simulink model "ES229A_HwTqCorrln"  (R2013b)
settings: Solver=FixedStepDiscrete  SolverMode=SingleTasking  StartTime=0.0  StopTime=1  FixedStep=0.002  RelTol=1e-3
undefined symbols (not defined in the file): ARCHGLBPRM_100MILLISEC_SEC_F32, FLTINJ_HWTQCORRLN_HWTQIDPTSIG, HwTqCorrlnChACmnModCmpLpFilActvnThd, HwTqCorrlnChACmnModCmpLpFilOutpLim, HwTqCorrlnChAImdtCorrlnChkFailThd, HwTqCorrlnChAImdtCorrlnChkPassThd, HwTqCorrlnChAStabStClrFltThd, HwTqCorrlnChAStabStSetFltThd, HwTqCorrlnChATqSumMaxLim, HwTqCorrlnChATraSumClrFltThd, HwTqCorrlnChATraSumSetFltThd, HwTqCorrlnChBCmnModCmpLpFilActvnThd, HwTqCorrlnChBCmnModCmpLpFilOutpLim, HwTqCorrlnChBImdtCorrlnChkFailThd, HwTqCorrlnChBImdtCorrlnChkPassThd, HwTqCorrlnChBStabStClrFltThd, HwTqCorrlnChBStabStSetFltThd, HwTqCorrlnChBTqSumMaxLim, HwTqCorrlnChBTraSumClrFltThd, HwTqCorrlnChBTraSumSetFltThd, HwTqCorrlnMaxStallTqA, HwTqCorrlnMaxStallTqB, HwTqCorrlnMaxStallTqC, HwTqCorrlnMaxStallTqD, HWTQSCA_CNT_U08, NtcNr1, NtcSts1, PARAMETERBYTE_CNT_U08, sigbuilder_block, SigQlfr1, STABSTLPFILSTVARIDELTALIM_HWNWTMTR_F32
libraries: simulink x25, Fil x12, NxtrLim x10, NxtrAbslt x6, FixdToFloat x2, FloatToFixdWithRound x2, LnrIntrpn x2, NxtrNvM x2
(part 1 of 4)
settings Model: Creator=nzy7l3  LastModifiedBy=CZ68DS
settings SolverCC: AutoInsertRateTranBlk=on  InsertRTBMode=Always
settings DataIOCC: LimitDataPoints=off  SaveFormat=Structure  ReturnWorkspaceOutputs=on
settings OptimizationCC: BlockReduction=off  InlineParams=on  ZeroExternalMemoryAtStartup=off  ZeroInternalMemoryAtStartup=off  OptimizeModelRefInitCode=on  LifeSpan=1
settings DebuggingCC: SignalInfNanChecking=error  SignalRangeChecking=warning  UnderspecifiedInitializationDetection=Simplified  MergeDetectMultiDrivingBlocksExec=error  SolverPrmCheckMsg=error  InheritedTsInSrcMsg=error  SingleTaskRateTransMsg=error  TasksWithSamePriorityMsg=error  SigSpecEnsureSampleTimeMsg=error  CheckMatrixSingularityMsg=error  ParameterUnderflowMsg=error  ParameterPrecisionLossMsg=error  ParameterTunabilityLossMsg=error  FixptConstUnderflowMsg=warning  FixptConstOverflowMsg=warning  VectorMatrixConversionMsg=error  SignalLabelMismatchMsg=error  UnconnectedInputMsg=error  UnconnectedOutputMsg=error  UnconnectedLineMsg=error  SFcnCompatibilityMsg=error  FrameProcessingCompatibilityMsg=error  UniqueDataStoreMsg=warning  BusObjectLabelMismatch=error  RootOutportRequireBusObject=error  AssertControl=DisableAll  ModelReferenceIOMsg=error  ModelReferenceVersionMismatchMessage=warning  ModelReferenceIOMismatchMessage=error  ModelReferenceDataLoggingMessage=error  StateNameClashWarn=warning  StrictBusMsg=ErrorOnBusTreatedAsVector  NonBusSignalsTreatedAsBus=error  SFUnexpectedBacktrackingDiag=error  SFInvalidInputDataAccessInChartInitDiag=error  SFNoUnconditionalDefaultTransitionDiag=error  SFTransitionOutsideNaturalParentDiag=error  SFUnconditionalTransitionShadowingDiag=error  SFUndirectedBroadcastEventsDiag=error
settings ModelReferenceCC: ModelReferenceNumInstancesAllowed=Single
settings RTWCC: SystemTargetFile=autosar.tlc  GenCodeOnly=on  TemplateMakefile=ert_default_tmf  Description=AUTOSAR  GenerateReport=on  LaunchReport=on
settings CodeAppCC: GenerateComments=off  IgnoreCustomStorageClasses=off  CustomSymbolStrType=$N$R$M  CustomSymbolStrBlkIO=$N$M  SimulinkBlockComments=off
settings STFCustomTargetCC: CodeReplacementLibrary=C89/C90 (ANSI)  ParMdlRefBuildCompliant=on  CompOptLevelCompliant=on  IncludeMdlTerminateFcn=off  CombineOutputUpdateFcns=on  SuppressErrorStatus=on  ERTFirstTimeCompliant=on  ERTCustomFileBanners=on  SupportNonFinite=off  SupportComplex=off  SupportContinuousTime=off  SupportNonInlinedSFcns=off  MATLABClassNameForMDSCustomization=Simulink.SoftwareTarget.ERTCustomization  AutosarCompliant=on  GRTInterface=off  SystemTargetFile=autosar.tlc
settings ERTTargetCC: CodeReplacementLibrary=C89/C90 (ANSI)  ConcurrentExecutionCompliant=off  IncludeMdlTerminateFcn=off  SuppressErrorStatus=on  SupportNonFinite=off  SupportComplex=off  ModelStepFunctionPrototypeControlCompliant=off  CPPClassGenCompliant=off  AutosarCompliant=on  InlinedParameterPlacement=NonHierarchical  ERTCustomFileTemplate=example_file_process.tlc  EnableUserReplacementTypes=on

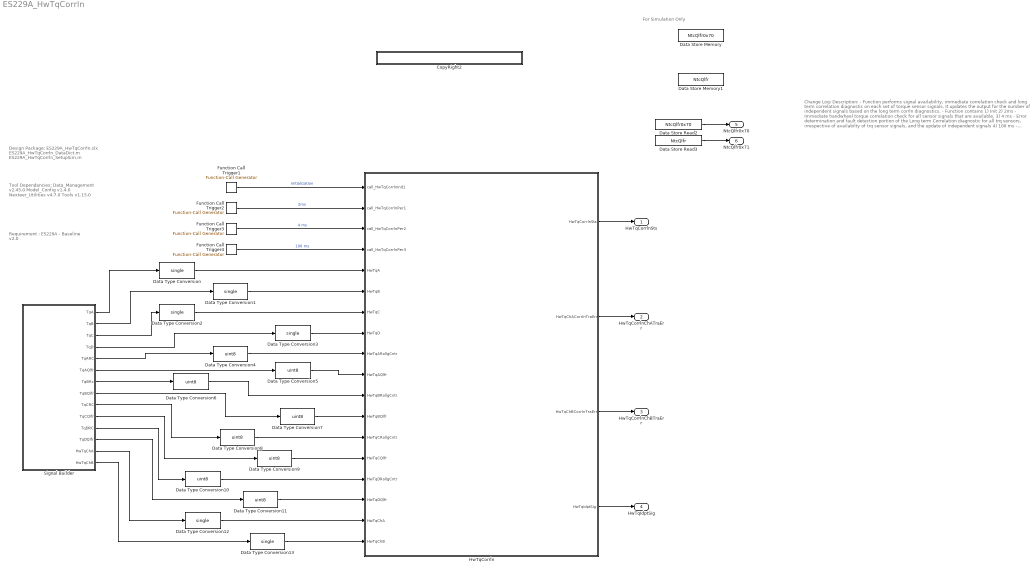
== system ES229A_HwTqCorrln ==
  note: Change Log:
      |
      | Description:
      | - Function performs signal availability, immediate correlation check and long term correlation diagnostic
      | on each set of torque sensor signals.
      | It updates the output for the number of independent signals based on the long term corrln diagnostics.
      | - Function contains
      | 1) Init
      | 2) 2ms - Immediate handwheel torque correlation check for all sensor signals that are available.
      | 3) 4 ms - Error determination and fault detection portion of the Long term Correlation diagnostic for all trq sensors,
      | irrespective of availabilty of trq sensor signals, and the update of independent signals
      | 4) 100 ms - Common mode long term compensation component of the Correlation diagnostic based on trimmed hw tq
      | derived from a pair of trq sensors.
      |
      | Copyright Blocks added to each layer
      |
      |
      | Rev: 3.2.0
      | Date:12OCT2016
      | Change Control #: EA4#8002
      | DRW: Keyur Patel
      | Description:
      | Code Impact:
      | - corrected FLTINJ_HWTQCORRLN_HWTQIDPTSIG as per DF001A
      |
      |
      | Rev: 3.1.0
      | Date:12SEPT2016
      | Change Control #: EA4#7556
      | DRW: Keyur Patel
      | Description:
      | Code Impact:
      | - Use     instead of FLTINJ_IDPTSIG_HWTQCORRLN in m file.
      |
      | Rev: 3.0.0
      | Date:28MAR2016
      | Change Control #: EA4#5051, EA4#5018
      | DRW: Praveen Devaraj / Muragesh Asundi (KPIT)
      | Description:
      | Code Impact:
      | - Two output variables HwTqChACorrlnTraErr and HwTqChBCorrlnTraErr have been added
      | -  Limit function is also added for these outputs
      | - Display variables 'dHwTqCorrlnChATraErr' and 'dHwTqCorrlnChBTraErr' have been deleted
      | No Code Impact:
      | - As per Anomaly  EA4#2139, model clean up is done function 'HwTqCorrlnInit1' to match code.
      | Color code:
      | - All changes are highlighted in red foreground color
      |
      | Rev: Synergy
      | Date:27OCT2015
      | Change Control #: EA4#2119
      | DRW: A.Amberkar
      | Description:
      | - Captured in WR comments - NtcNr2 revise to NtcNr1 and use LimDyn_f32 library block.
      | - For anomaly#2139 to prepare model for MIL testing - removed delay blocks in Signal availability
      | and replaced with already defined PIM data.
      |
      | Rev: Synergy
      | Date:01OCT2015
      | Change Control #: EA4#1347
      | DRW: A.Amberkar
      | Description:
      | - Captured in WR comments - new immdt corrln check, limit on SS LPF, new independent signals truth table
      |
      | Rev: Synergy
      | Date: 11AUG2015
      | Change Control #:EA4#1273
      | DRW: A.Amberkar
      | Description:
      | - Changes to match code - captured in WR comments
      |
      | Rev: Synergy
      | Date: 13JUL2015
      | Change Control #:EA4#768
      | DRW: A.Amberkar
      | Description:
      | - Initial Release
      |
      | Rev: Synergy
      | Date: 17JUN2015
      | Change Control #: EA4#768
      | DRW: Aparna Amberkar
  note: Design Package:
      | ES229A_HwTqCorrln.slx
      | ES229A_HwTqCorrln_DataDict.m
      | ES229A_HwTqCorrln_SetupSim.m
  note: Tool Dependancies:
      |
      | Data_Management v2.45.0
      | Model_Config v1.4.0
      | Nexteer_Utilities v4.7.0
      | Tools v1.15.0
  note: Requirement :
      |
      | ES229A - Baseline v2.0
  note: For Simulation Only
  CopyRight2 : Subsystem  Description=|  mask(Copyright Information){none=on}
      | Copyright info block.                                               
      |                                                                     
      | Place copyright information at the top of every subsystem in design.
      mask prompts: none "No parameters"
      mask help: Place copyright information at the top of every subsystem in design.
      mask Display:
      | NxtrConf = 'Nexteer Confidential';
      | 
      | sys = bdroot; %handle for the current model ("system")
      | first = get_param(sys,'Created');
      | first = first(end-3:end);  %year is last four digits
      | 
      | last = get_param(sys,'LastModifiedDate');
      | if isempty(last)
      |     last = datestr(now,'yyyy');
      | else
      |     last = last(end-3:end);
      | end
      | 
      | if strcmp(first,last)
      |     fprintf('%s -- Copyright %s Nexteer',NxtrConf,first)
      | else
      |     fprintf('%s -- %s%s- %s Nexteer',NxtrConf,char(169),first,last)
      | end
  Data Store Read2 : DataStoreRead  DataStoreName=NtcQlfr0x70  SampleTime=.002
  Data Store Read3 : DataStoreRead  DataStoreName=NtcQlfr  SampleTime=.002
  Data Store Memory : DataStoreMemory  DataStoreName=NtcQlfr0x70  ReadBeforeWriteMsg=warning  WriteAfterWriteMsg=warning  WriteAfterReadMsg=warning  OutDataTypeStr=uint8
      settings: AttributesFormatString=|
      | Simulation Purpose Only.
      | Do Not Code this block
      | Diagnostic Manager Owns this requirement
  Data Store Memory1 : DataStoreMemory  DataStoreName=NtcQlfr  ReadBeforeWriteMsg=warning  WriteAfterWriteMsg=warning  WriteAfterReadMsg=warning  OutDataTypeStr=uint8
      settings: AttributesFormatString=|
      | Simulation Purpose Only.
      | Do Not Code this block
      | Diagnostic Manager Owns this requirement
  Data Type Conversion{,1..3,12..13} (6 alike) : DataTypeConversion  OutDataTypeStr=single
  Data Type Conversion{4..11} (8 alike) : DataTypeConversion  OutDataTypeStr=uint8
  Function Call Trigger{1..4} (4 alike) : simulink/Ports & Subsystems/Function-Call Generator  sample_time=.002  numberOfIterations=1
  HwTqCorrln : Subsystem
  Signal Builder : Subsystem  Tag=STV Subsys  LoadFcn=sigbuilder_block('load');  StartFcn=sigbuilder_block('start');  StopFcn=sigbuilder_block('stop');  ClipboardFcn=sigbuilder_block('clipboard');  mask(Sigbuilder block){}
      mask help: Simulink:masks:SigbuilderBlock_MD
      mask init:
      | if ~strcmp(get_param(bdroot(gcbh),'SimulationStatus'),'stopped') tuvar = sigbuilder_block('maskInit'); end
      settings: CopyFcn=sigbuilder_block('copy');  DeleteFcn=sigbuilder_block('delete');  ModelCloseFcn=sigbuilder_block('modelClose');  PreSaveFcn=sigbuilder_block('preSave');  PauseFcn=sigbuilder_block('pause');  ContinueFcn=sigbuilder_block('continue');  NameChangeFcn=sigbuilder_block('namechange');  OpenFcn=sigbuilder_block('open',[5.58621 28.5517 1009.24 486 ]);  CloseFcn=sigbuilder_block('close');
      mask Display: plot(0, 0, 100, 100,[2, 2, 32, 32, 2], [68, 8, 8, 68, 68],[32, 2], [38, 38], [32, 19, 2],[53, 60, 44], [32, 17, 17, 2],[16, 16, 31, 31]);txt = getActiveGroup(gcbh);text(2, 100, txt,'verticalAlignment', 'top');
  HwTqCorrlnSts : Outport
  HwTqCorrlnChATraErr : Outport  Port=2
  HwTqCorrlnChBTraErr : Outport  Port=3
  HwTqIdptSig : Outport  Port=4
  NtcQlfr0x70 : Outport  Port=5
  NtcQlfr0x71 : Outport  Port=6
  wires:
  Function Call Trigger1/1 -> HwTqCorrln/1(call_HwTqCorrlnInit1)  "Initialization"
  Function Call Trigger3/1 -> HwTqCorrln/3("call_HwTqCorrlnPer2 ")  "4 ms"
  Function Call Trigger2/1 -> HwTqCorrln/2(call_HwTqCorrlnPer1)  "2ms"
  Function Call Trigger4/1 -> HwTqCorrln/4(call_HwTqCorrlnPer3)  "100 ms"
  Signal Builder/13(HwTqChA) -> Data Type Conversion12/1
  Signal Builder/14(HwTqChB) -> Data Type Conversion13/1
  Data Type Conversion/1 -> HwTqCorrln/5(HwTqA)
  Data Type Conversion1/1 -> HwTqCorrln/6(HwTqB)
  Signal Builder/3(TqC) -> Data Type Conversion2/1
  Signal Builder/5(TqARC) -> Data Type Conversion4/1
  Signal Builder/6(TqAQlfr) -> Data Type Conversion5/1
  Signal Builder/7(TqBRc) -> Data Type Conversion6/1
  Signal Builder/8(TqBQlfr) -> Data Type Conversion7/1
  Signal Builder/9(TqCRC) -> Data Type Conversion8/1
  Signal Builder/10(TqCQlfr) -> Data Type Conversion9/1
  Signal Builder/11(TqDRC) -> Data Type Conversion10/1
  Signal Builder/12(TqDQlfr) -> Data Type Conversion11/1
  Data Type Conversion2/1 -> HwTqCorrln/7(HwTqC)
  Data Type Conversion3/1 -> HwTqCorrln/8(HwTqD)
  Data Type Conversion4/1 -> HwTqCorrln/9(HwTqARollgCntr)
  Data Type Conversion5/1 -> HwTqCorrln/10(HwTqAQlfr)
  Data Type Conversion6/1 -> HwTqCorrln/11(HwTqBRollgCntr)
  Data Type Conversion7/1 -> HwTqCorrln/12(HwTqBQlfr)
  Data Type Conversion8/1 -> HwTqCorrln/13(HwTqCRollgCntr)
  Data Type Conversion9/1 -> HwTqCorrln/14(HwTqCQlfr)
  Data Type Conversion10/1 -> HwTqCorrln/15(HwTqDRollgCntr)
  Data Type Conversion11/1 -> HwTqCorrln/16(HwTqDQlfr)
  Data Type Conversion12/1 -> HwTqCorrln/17(HwTqChA)
  Data Type Conversion13/1 -> HwTqCorrln/18(HwTqChB)
  Signal Builder/1(TqA) -> Data Type Conversion/1
  Signal Builder/2(TqB) -> Data Type Conversion1/1
  Signal Builder/4(TqD) -> Data Type Conversion3/1
  HwTqCorrln/1(HwTqCorrlnSts) -> HwTqCorrlnSts/1
  HwTqCorrln/4(HwTqIdptSig) -> HwTqIdptSig/1
  HwTqCorrln/3(HwTqChBCorrlnTraErr) -> HwTqCorrlnChBTraErr/1
  HwTqCorrln/2(HwTqChACorrlnTraErr) -> HwTqCorrlnChATraErr/1
  Data Store Read2/1 -> NtcQlfr0x70/1
  Data Store Read3/1 -> NtcQlfr0x71/1

== system ES229A_HwTqCorrln/CopyRight2 ==

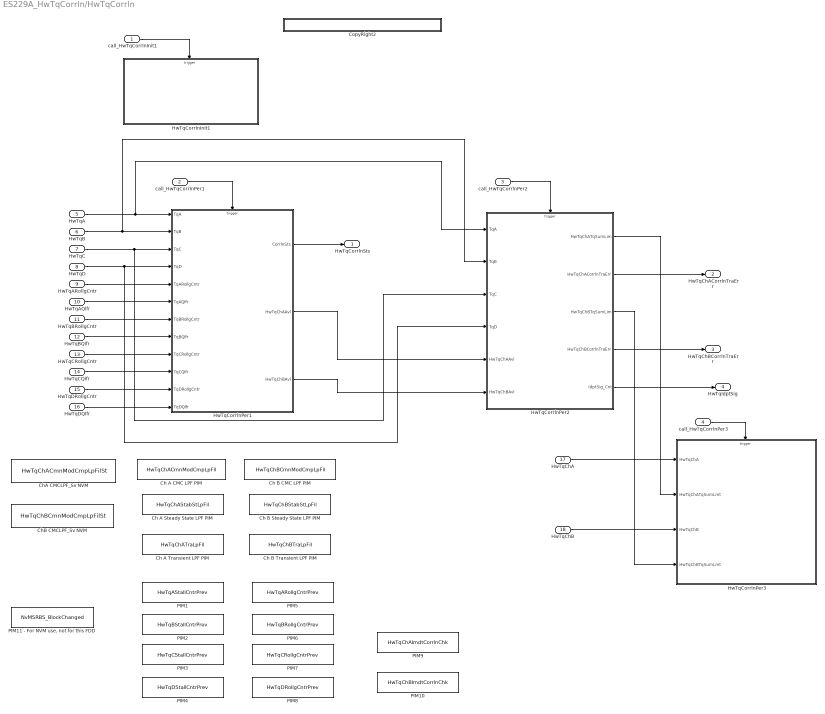
== system ES229A_HwTqCorrln/HwTqCorrln ==
  call_HwTqCorrlnInit1 : Inport
  call_HwTqCorrlnPer1 : Inport  Port=2
  "call_HwTqCorrlnPer2 " : Inport  Port=3
  call_HwTqCorrlnPer3 : Inport  Port=4
  HwTqA : Inport  Port=5
  HwTqB : Inport  Port=6
  HwTqC : Inport  Port=7
  HwTqD : Inport  Port=8
  HwTqARollgCntr : Inport  Port=9
  HwTqAQlfr : Inport  Port=10
  HwTqBRollgCntr : Inport  Port=11
  HwTqBQlfr : Inport  Port=12
  HwTqCRollgCntr : Inport  Port=13
  HwTqCQlfr : Inport  Port=14
  HwTqDRollgCntr : Inport  Port=15
  HwTqDQlfr : Inport  Port=16
  HwTqChA : Inport  Port=17
  HwTqChB : Inport  Port=18
  " PIM1" : DataStoreMemory  DataStoreName=HwTqAStallCntrPrev  ReadBeforeWriteMsg=warning  WriteAfterWriteMsg=warning  WriteAfterReadMsg=warning  StateMustResolveToSignalObject=on
  " PIM11 - For NVM use, not for this FDD" : DataStoreMemory  DataStoreName=NvMSRBS_BlockChanged  ReadBeforeWriteMsg=warning  WriteAfterWriteMsg=warning  WriteAfterReadMsg=warning
  " PIM2" : DataStoreMemory  DataStoreName=HwTqBStallCntrPrev  ReadBeforeWriteMsg=warning  WriteAfterWriteMsg=warning  WriteAfterReadMsg=warning  StateMustResolveToSignalObject=on
  " PIM3" : DataStoreMemory  DataStoreName=HwTqCStallCntrPrev  ReadBeforeWriteMsg=warning  WriteAfterWriteMsg=warning  WriteAfterReadMsg=warning  StateMustResolveToSignalObject=on
  " PIM4" : DataStoreMemory  DataStoreName=HwTqDStallCntrPrev  ReadBeforeWriteMsg=warning  WriteAfterWriteMsg=warning  WriteAfterReadMsg=warning  StateMustResolveToSignalObject=on
  " PIM5" : DataStoreMemory  DataStoreName=HwTqARollgCntrPrev  ReadBeforeWriteMsg=warning  WriteAfterWriteMsg=warning  WriteAfterReadMsg=warning  StateMustResolveToSignalObject=on
  " PIM6" : DataStoreMemory  DataStoreName=HwTqBRollgCntrPrev  ReadBeforeWriteMsg=warning  WriteAfterWriteMsg=warning  WriteAfterReadMsg=warning  StateMustResolveToSignalObject=on
  " PIM7" : DataStoreMemory  DataStoreName=HwTqCRollgCntrPrev  ReadBeforeWriteMsg=warning  WriteAfterWriteMsg=warning  WriteAfterReadMsg=warning  StateMustResolveToSignalObject=on
  " PIM8" : DataStoreMemory  DataStoreName=HwTqDRollgCntrPrev  ReadBeforeWriteMsg=warning  WriteAfterWriteMsg=warning  WriteAfterReadMsg=warning  StateMustResolveToSignalObject=on
  " PIM9" : DataStoreMemory  DataStoreName=HwTqChAImdtCorrlnChk  ReadBeforeWriteMsg=warning  WriteAfterWriteMsg=warning  WriteAfterReadMsg=warning  StateMustResolveToSignalObject=on
  Ch A CMC LPF PIM : DataStoreMemory  RequirementInfo="{'linktype_rmi_doors' '0000c477 (/ESG Group/FDD Module Requirements/EA4 Specific/ES229A_HwTqCorrln)' '#ES229A_123' 'true' 'REQ:  ES229A_123' '' } %GIDa_6766c665_50e1_4b65_9ecd_d704019af802"  DataStoreName=HwTqChACmnModCmpLpFil  ReadBeforeWriteMsg=warning  WriteAfterWriteMsg=warning  WriteAfterReadMsg=warning  InitialValue=struct('FilSt',single(0),'FilGain',single(0))  OutDataTypeStr=Bus: FilLpRec1  StateMustResolveToSignalObject=on
  Ch A Steady State LPF PIM : DataStoreMemory  RequirementInfo="{'linktype_rmi_doors' '0000c477 (/ESG Group/FDD Module Requirements/EA4 Specific/ES229A_HwTqCorrln)' '#ES229A_118' 'true' 'REQ:  ES229A_118' '' } %GIDa_9e19175a_f7a8_42e9_9550_54226049f41b"  DataStoreName=HwTqChAStabStLpFil  ReadBeforeWriteMsg=warning  WriteAfterWriteMsg=warning  WriteAfterReadMsg=warning  InitialValue=struct('FilSt',single(0),'FilGain',single(0))  OutDataTypeStr=Bus: FilLpRec1  StateMustResolveToSignalObject=on
  Ch A Transient LPF PIM : DataStoreMemory  RequirementInfo="{'linktype_rmi_doors' '0000c477 (/ESG Group/FDD Module Requirements/EA4 Specific/ES229A_HwTqCorrln)' '#ES229A_117' 'true' 'REQ:  ES229A_117' '' } %GIDa_8850e544_67f8_4526_8ea6_263e9ece6630"  DataStoreName=HwTqChATraLpFil  ReadBeforeWriteMsg=warning  WriteAfterWriteMsg=warning  WriteAfterReadMsg=warning  InitialValue=struct('FilSt',single(0),'FilGain',single(0))  OutDataTypeStr=Bus: FilLpRec1  StateMustResolveToSignalObject=on
  Ch B CMC LPF PIM : DataStoreMemory  RequirementInfo="{'linktype_rmi_doors' '0000c477 (/ESG Group/FDD Module Requirements/EA4 Specific/ES229A_HwTqCorrln)' '#ES229A_133' 'true' 'REQ:  ES229A_133' '' } %GIDa_5dd4475c_8cba_4d1f_98d6_68220c356134"  DataStoreName=HwTqChBCmnModCmpLpFil  ReadBeforeWriteMsg=warning  WriteAfterWriteMsg=warning  WriteAfterReadMsg=warning  InitialValue=struct('FilSt',single(0),'FilGain',single(0))  OutDataTypeStr=Bus: FilLpRec1  StateMustResolveToSignalObject=on
  Ch B Steady State LPF PIM : DataStoreMemory  RequirementInfo="{'linktype_rmi_doors' '0000c477 (/ESG Group/FDD Module Requirements/EA4 Specific/ES229A_HwTqCorrln)' '#ES229A_132' 'true' 'REQ:  ES229A_132' '' } %GIDa_17cd5088_b902_4a38_b561_38fb02043e47"  DataStoreName=HwTqChBStabStLpFil  ReadBeforeWriteMsg=warning  WriteAfterWriteMsg=warning  WriteAfterReadMsg=warning  InitialValue=struct('FilSt',single(0),'FilGain',single(0))  OutDataTypeStr=Bus: FilLpRec1  StateMustResolveToSignalObject=on
  Ch B Transient LPF PIM : DataStoreMemory  RequirementInfo="{'linktype_rmi_doors' '0000c477 (/ESG Group/FDD Module Requirements/EA4 Specific/ES229A_HwTqCorrln)' '#ES229A_131' 'true' 'REQ:  ES229A_131' '' } %GIDa_8ffac466_7c6f_4ce2_8da4_58b961cf122e"  DataStoreName=HwTqChBTraLpFil  ReadBeforeWriteMsg=warning  WriteAfterWriteMsg=warning  WriteAfterReadMsg=warning  InitialValue=struct('FilSt',single(0),'FilGain',single(0))  OutDataTypeStr=Bus: FilLpRec1  StateMustResolveToSignalObject=on
  "ChA CMCLPF_Sv NVM " : DataStoreMemory  RequirementInfo="{'linktype_rmi_doors' '0000c477 (/ESG Group/FDD Module Requirements/EA4 Specific/ES229A_HwTqCorrln)' '#ES229A_108' 'true' 'REQ:  ES229A_108' '' } %GIDa_3034ba17_e21f_4c4f_92c6_2686ce98dd15"  DataStoreName=HwTqChACmnModCmpLpFilSt  ReadBeforeWriteMsg=warning  WriteAfterWriteMsg=warning  WriteAfterReadMsg=warning  StateMustResolveToSignalObject=on
  ChB CMCLPF_Sv NVM : DataStoreMemory  RequirementInfo="{'linktype_rmi_doors' '0000c477 (/ESG Group/FDD Module Requirements/EA4 Specific/ES229A_HwTqCorrln)' '#ES229A_109' 'true' 'REQ:  ES229A_109' '' } %GIDa_0d493052_0847_4007_805a_59667ab2ab4a"  DataStoreName=HwTqChBCmnModCmpLpFilSt  ReadBeforeWriteMsg=warning  WriteAfterWriteMsg=warning  WriteAfterReadMsg=warning  StateMustResolveToSignalObject=on
  CopyRight2 : Subsystem  Description=|  mask(Copyright Information){none=on}
      | Copyright info block.                                               
      |                                                                     
      | Place copyright information at the top of every subsystem in design.
      mask prompts: none "No parameters"
      mask help: Place copyright information at the top of every subsystem in design.
      mask Display:
      | NxtrConf = 'Nexteer Confidential';
      | 
      | sys = bdroot; %handle for the current model ("system")
      | first = get_param(sys,'Created');
      | first = first(end-3:end);  %year is last four digits
      | 
      | last = get_param(sys,'LastModifiedDate');
      | if isempty(last)
      |     last = datestr(now,'yyyy');
      | else
      |     last = last(end-3:end);
      | end
      | 
      | if strcmp(first,last)
      |     fprintf('%s -- Copyright %s Nexteer',NxtrConf,first)
      | else
      |     fprintf('%s -- %s%s- %s Nexteer',NxtrConf,char(169),first,last)
      | end
  HwTqCorrlnInit1 : Subsystem  TreatAsAtomicUnit=on
  HwTqCorrlnPer1 : Subsystem  RequirementInfo={} %GIDa_553bcabc_51d1_46d6_b172_9c866a2e5d81  TreatAsAtomicUnit=on
  HwTqCorrlnPer2 : Subsystem  RequirementInfo={} %GIDa_3a71e2f5_a14f_415b_8a15_f21caafb563d  TreatAsAtomicUnit=on
  HwTqCorrlnPer3 : Subsystem  TreatAsAtomicUnit=on
  PIM10 : DataStoreMemory  DataStoreName=HwTqChBImdtCorrlnChk  ReadBeforeWriteMsg=warning  WriteAfterWriteMsg=warning  WriteAfterReadMsg=warning  StateMustResolveToSignalObject=on
  HwTqCorrlnSts : Outport
  HwTqChACorrlnTraErr : Outport  RequirementInfo={'linktype_rmi_doors' '0000c477 (/ESG Group/FDD Module Requirements/EA4 Specific/ES229A_HwTqCorrln)' '#ES229A_165' 'true' 'REQ: ES229A_165' '' } %GIDa_67389848_7ddc_4db7_86e8_1b151ddb89f7  Port=2
  HwTqChBCorrlnTraErr : Outport  RequirementInfo={'linktype_rmi_doors' '0000c477 (/ESG Group/FDD Module Requirements/EA4 Specific/ES229A_HwTqCorrln)' '#ES229A_166' 'true' 'REQ: ES229A_166' '' } %GIDa_a2392685_2b71_4620_85c8_5b6a06a62cb6  Port=3
  HwTqIdptSig : Outport  Port=4
  wires:
  call_HwTqCorrlnInit1/1 -> HwTqCorrlnInit1/Trigger
  call_HwTqCorrlnPer1/1 -> HwTqCorrlnPer1/Trigger
  "call_HwTqCorrlnPer2 "/1 -> HwTqCorrlnPer2/Trigger
  HwTqCorrlnPer1/1(CorrlnSts) -> HwTqCorrlnSts/1
  call_HwTqCorrlnPer3/1 -> HwTqCorrlnPer3/Trigger
  HwTqCorrlnPer2/5(IdptSig_Cnt) -> HwTqIdptSig/1
  HwTqCorrlnPer2/1(HwTqChATqSumLim) -> HwTqCorrlnPer3/2(HwTqChATqSumLmt)
  HwTqChA/1 -> HwTqCorrlnPer3/1(HwTqChA)
  HwTqChB/1 -> HwTqCorrlnPer3/3(HwTqChB)
  HwTqAQlfr/1 -> HwTqCorrlnPer1/6(TqAQlfr)
  HwTqA/1 -> HwTqCorrlnPer2/1(TqA), HwTqCorrlnPer1/1(TqA)
  HwTqB/1 -> HwTqCorrlnPer2/2(TqB), HwTqCorrlnPer1/2(TqB)
  HwTqC/1 -> HwTqCorrlnPer1/3(TqC), HwTqCorrlnPer2/3(TqC)
  HwTqD/1 -> HwTqCorrlnPer2/4(TqD), HwTqCorrlnPer1/4(TqD)
  HwTqARollgCntr/1 -> HwTqCorrlnPer1/5(TqARollgCntr)
  HwTqBRollgCntr/1 -> HwTqCorrlnPer1/7(TqBRollgCntr)
  HwTqBQlfr/1 -> HwTqCorrlnPer1/8(TqBQlfr)
  HwTqCRollgCntr/1 -> HwTqCorrlnPer1/9(TqCRollgCntr)
  HwTqCQlfr/1 -> HwTqCorrlnPer1/10(TqCQlfr)
  HwTqDRollgCntr/1 -> HwTqCorrlnPer1/11(TqDRollgCntr)
  HwTqDQlfr/1 -> HwTqCorrlnPer1/12(TqDQlfr)
  HwTqCorrlnPer2/3(HwTqChBTqSumLim) -> HwTqCorrlnPer3/4(HwTqChBTqSumLmt)
  HwTqCorrlnPer1/2(HwTqChAAvl) -> HwTqCorrlnPer2/5(HwTqChAAvl)
  HwTqCorrlnPer1/3(HwTqChBAvl) -> HwTqCorrlnPer2/6(HwTqChBAvl)
  HwTqCorrlnPer2/2(HwTqChACorrlnTraErr) -> HwTqChACorrlnTraErr/1
  HwTqCorrlnPer2/4(HwTqChBCorrlnTraErr) -> HwTqChBCorrlnTraErr/1

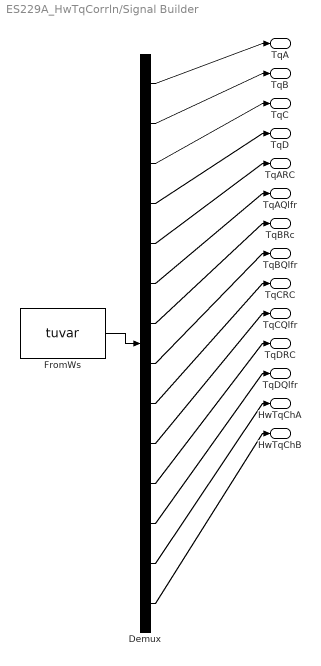
== system ES229A_HwTqCorrln/Signal Builder ==
  Demux : Demux  Tag=STV Demux  Outputs=14
  FromWs : FromWorkspace  Tag=STV FromWs  VariableName=tuvar  SampleTime=0
      SigBuilderData=|
      | common.afterFinalStr = 'Extrapolate'
      | common.sampleTime = 0
      | dataSet(1).timeRange = [0 5]
      | dataSet(1).name = 'HwTq Ideal Inputs'
      | dataSet(2).timeRange = [0 5]
      | dataSet(2).name = 'HwTqB Value Offset Fault'
      | dataSet(3).timeRange = [0 5]
      | dataSet(3).name = 'HwTqA RC Fault'
      | dataSet(4).timeRange = [0 5]
      | dataSet(4).name = 'HwTqA Qlfr Fault'
      | dataSet(5).timeRange = [0 5]
      | dataSet(5).name = 'HwTqA Corrln and Avl Fault'
      | sbobj.Groups(1).Name = 'HwTq Ideal Inputs'
      | sbobj.Groups(1).Signals(1).Name = 'TqA'
      | sbobj.Groups(1).Signals(1).XData = [0 1 1 2 2 3 3 4 4 5]
      | sbobj.Groups(1).Signals(1).YData = [-10 10 -10 10 -10 10 -10 10 -10 10]
      | sbobj.Groups(1).Signals(2).Name = 'TqB'
      | sbobj.Groups(1).Signals(2).XData = [0 1 1 2 2 3 3 4 4 5]
      | sbobj.Groups(1).Signals(2).YData = [-10 10 -10 10 -10 10 -10 10 -10 10]
      | sbobj.Groups(1).Signals(3).Name = 'TqC'
      | sbobj.Groups(1).Signals(3).XData = [0 1 1 2 2 3 3 4 4 5]
      | sbobj.Groups(1).Signals(3).YData = [-10 10 -10 10 -10 10 -10 10 -10 10]
      | sbobj.Groups(1).Signals(4).Name = 'TqD'
      | sbobj.Groups(1).Signals(4).XData = [0 1 1 2 2 3 3 4 4 5]
      | sbobj.Groups(1).Signals(4).YData = [-10 10 -10 10 -10 10 -10 10 -10 10]
      | sbobj.Groups(1).Signals(5).Name = 'TqARC'
      | sbobj.Groups(1).Signals(5).XData = [0 1 1 2 2 3 3 4 4 5]
      | sbobj.Groups(1).Signals(5).YData = [-1 255 -1 255 -1 255 -1 255 -1 255]
      | sbobj.Groups(1).Signals(6).Name = 'TqAQlfr'
      | sbobj.Groups(1).Signals(6).XData = [0 5]
      | sbobj.Groups(1).Signals(6).YData = [1 1]
      | sbobj.Groups(1).Signals(7).Name = 'TqBRc'
      | sbobj.Groups(1).Signals(7).XData = [0 1 1 2 2 3 3 4 4 5]
      | sbobj.Groups(1).Signals(7).YData = [-1 255 -1 255 -1 255 -1 255 -1 255]
      | sbobj.Groups(1).Signals(8).Name = 'TqBQlfr'
      | sbobj.Groups(1).Signals(8).XData = [0 5]
      | sbobj.Groups(1).Signals(8).YData = [1 1]
      | sbobj.Groups(1).Signals(9).Name = 'TqCRC'
      | sbobj.Groups(1).Signals(9).XData = [0 1 1 2 2 3 3 4 4 5]
      | sbobj.Groups(1).Signals(9).YData = [-1 255 -1 255 -1 255 -1 255 -1 255]
      | sbobj.Groups(1).Signals(10).Name = 'TqCQlfr'
      | sbobj.Groups(1).Signals(10).XData = [0 5]
      | sbobj.Groups(1).Signals(10).YData = [1 1]
      | sbobj.Groups(1).Signals(11).Name = 'TqDRC'
      | sbobj.Groups(1).Signals(11).XData = [0 1 1 2 2 3 3 4 4 5]
      | sbobj.Groups(1).Signals(11).YData = [-1 255 -1 255 -1 255 -1 255 -1 255]
      | sbobj.Groups(1).Signals(12).Name = 'TqDQlfr'
      | sbobj.Groups(1).Signals(12).XData = [0 5]
      | sbobj.Groups(1).Signals(12).YData = [1 1]
      | sbobj.Groups(1).Signals(13).Name = 'HwTqChA'
      | sbobj.Groups(1).Signals(13).XData = [0 1 1 2 2 3 3 4 4 5]
      | sbobj.Groups(1).Signals(13).YData = [-10 10 -10 10 -10 10 -10 10 -10 10]
      | sbobj.Groups(1).Signals(14).Name = 'HwTqChB'
      | sbobj.Groups(1).Signals(14).XData = [0 1 1 2 2 3 3 4 4 5]
      | sbobj.Groups(1).Signals(14).YData = [-10 10 -10 10 -10 10 -10 10 -10 10]
      | sbobj.Groups(1).TimeRange = [0 5]
      | sbobj.Groups(2).Name = 'HwTqB Value Offset Fault'
      | sbobj.Groups(2).Signals(1).Name = 'TqA'
      | sbobj.Groups(2).Signals(1).XData = [0 1 1 2 2 3 3 4 4 5]
      | sbobj.Groups(2).Signals(1).YData = [-10 10 -10 10 -10 10 -10 10 -10 10]
      | sbobj.Groups(2).Signals(2).Name = 'TqB'
      | sbobj.Groups(2).Signals(2).XData = [0 1 2 2 3 3 4 4 5]
      | sbobj.Groups(2).Signals(2).YData = [0 -1 0 -10 10 -10 10 -10 10]
      | sbobj.Groups(2).Signals(3).Name = 'TqC'
      | sbobj.Groups(2).Signals(3).XData = [0 1 1 2 2 3 3 4 4 5]
      | sbobj.Groups(2).Signals(3).YData = [-10 10 -10 10 -10 10 -10 10 -10 10]
      | sbobj.Groups(2).Signals(4).Name = 'TqD'
      | sbobj.Groups(2).Signals(4).XData = [0 1 1 2 2 3 3 4 4 5]
      | sbobj.Groups(2).Signals(4).YData = [-10 10 -10 10 -10 10 -10 10 -10 10]
      | sbobj.Groups(2).Signals(5).Name = 'TqARC'
      | sbobj.Groups(2).Signals(5).XData = [0 1 1 2 2 3 3 4 4 5]
      | sbobj.Groups(2).Signals(5).YData = [-1 255 -1 255 -1 255 -1 255 -1 255]
      | sbobj.Groups(2).Signals(6).Name = 'TqAQlfr'
      | sbobj.Groups(2).Signals(6).XData = [0 5]
      | sbobj.Groups(2).Signals(6).YData = [1 1]
      | sbobj.Groups(2).Signals(7).Name = 'TqBRc'
      | sbobj.Groups(2).Signals(7).XData = [0 1 1 2 2 3 3 4 4 5]
      | sbobj.Groups(2).Signals(7).YData = [-1 255 -1 255 -1 255 -1 255 -1 255]
      | sbobj.Groups(2).Signals(8).Name = 'TqBQlfr'
      | sbobj.Groups(2).Signals(8).XData = [0 5]
      | sbobj.Groups(2).Signals(8).YData = [1 1]
      | sbobj.Groups(2).Signals(9).Name = 'TqCRC'
      | sbobj.Groups(2).Signals(9).XData = [0 1 1 2 2 3 3 4 4 5]
      | sbobj.Groups(2).Signals(9).YData = [-1 255 -1 255 -1 255 -1 255 -1 255]
      | sbobj.Groups(2).Signals(10).Name = 'TqCQlfr'
      | sbobj.Groups(2).Signals(10).XData = [0 5]
      | sbobj.Groups(2).Signals(10).YData = [1 1]
      | sbobj.Groups(2).Signals(11).Name = 'TqDRC'
      | sbobj.Groups(2).Signals(11).XData = [0 1 1 2 2 3 3 4 4 5]
      | sbobj.Groups(2).Signals(11).YData = [-1 255 -1 255 -1 255 -1 255 -1 255]
      | sbobj.Groups(2).Signals(12).Name = 'TqDQlfr'
      | sbobj.Groups(2).Signals(12).XData = [0 5]
      | sbobj.Groups(2).Signals(12).YData = [1 1]
      | sbobj.Groups(2).Signals(13).Name = 'HwTqChA'
      | sbobj.Groups(2).Signals(13).XData = [0 1 1 2 2 3 3 4 4 5 5]
      | sbobj.Groups(2).Signals(13).YData = [-10 10 -10 10 -10 10 -10 10 -10 10 -10]
      | sbobj.Groups(2).Signals(14).Name = 'HwTqChB'
      | sbobj.Groups(2).Signals(14).XData = [0 1 1 2 2 3 3 4 4 5 5]
      | sbobj.Groups(2).Signals(14).YData = [-10 10 -10 10 -10 10 -10 10 -10 10 -10]
      | sbobj.Groups(2).TimeRange = [0 5]
      | sbobj.Groups(3).Name = 'HwTqA RC Fault'
      | sbobj.Groups(3).Signals(1).Name = 'TqA'
      | sbobj.Groups(3).Signals(1).XData = [0 1 1 2 2 3 3 4 4 5]
      | sbobj.Groups(3).Signals(1).YData = [-10 10 -10 10 -10 10 -10 10 -10 10]
      | sbobj.Groups(3).Signals(2).Name = 'TqB'
      | sbobj.Groups(3).Signals(2).XData = [0 0.5 1 1 1.5 2 2 2.5 3 3.5 4 4 4.5 5]
      | sbobj.Groups(3).Signals(2).YData = [-10 10 9 -10 0 10 -10 0 0 0 10 -10 0 10]
      | sbobj.Groups(3).Signals(3).Name = 'TqC'
      | sbobj.Groups(3).Signals(3).XData = [0 1 1 2 2 3 3 4 4 5]
      | sbobj.Groups(3).Signals(3).YData = [-10 10 -10 10 -10 10 -10 10 -10 10]
      | sbobj.Groups(3).Signals(4).Name = 'TqD'
      | sbobj.Groups(3).Signals(4).XData = [0 1 1 2 2 3 3 4 4 5]
      | sbobj.Groups(3).Signals(4).YData = [-10 10 -10 10 -10 10 -10 10 -10 10]
      | sbobj.Groups(3).Signals(5).Name = 'TqARC'
      | sbobj.Groups(3).Signals(5).XData = [0 0.5 1 1 1.5 1.5 2 2 2.5 2.5 3 3.5 4 4 5]
      | sbobj.Groups(3).Signals(5).YData = [0 200 200 0 200 0 200 0 200 0 0 0 200 0 200]
      | sbobj.Groups(3).Signals(6).Name = 'TqAQlfr'
      | sbobj.Groups(3).Signals(6).XData = [0 5]
      | sbobj.Groups(3).Signals(6).YData = [1 1]
      | sbobj.Groups(3).Signals(7).Name = 'TqBRc'
      | sbobj.Groups(3).Signals(7).XData = [0 1 1 2 2 3 3 4 4 5]
      | sbobj.Groups(3).Signals(7).YData = [-1 255 -1 255 -1 255 -1 255 -1 255]
      | sbobj.Groups(3).Signals(8).Name = 'TqBQlfr'
      | sbobj.Groups(3).Signals(8).XData = [0 5]
      | sbobj.Groups(3).Signals(8).YData = [1 1]
      | sbobj.Groups(3).Signals(9).Name = 'TqCRC'
      | sbobj.Groups(3).Signals(9).XData = [0 1 1 2 2 3 3 4 4 5]
      | sbobj.Groups(3).Signals(9).YData = [-1 255 -1 255 -1 255 -1 255 -1 255]
      | sbobj.Groups(3).Signals(10).Name = 'TqCQlfr'
      | sbobj.Groups(3).Signals(10).XData = [0 5]
      | sbobj.Groups(3).Signals(10).YData = [1 1]
      | sbobj.Groups(3).Signals(11).Name = 'TqDRC'
      | sbobj.Groups(3).Signals(11).XData = [0 1 1 2 2 3 3 4 4 5]
      | sbobj.Groups(3).Signals(11).YData = [-1 255 -1 255 -1 255 -1 255 -1 255]
      | sbobj.Groups(3).Signals(12).Name = 'TqDQlfr'
      | sbobj.Groups(3).Signals(12).XData = [0 5]
      | sbobj.Groups(3).Signals(12).YData = [1 1]
      | sbobj.Groups(3).Signals(13).Name = 'HwTqChA'
      | sbobj.Groups(3).Signals(13).XData = [0 1 1 2 2 3 3 4 4 5 5]
      | sbobj.Groups(3).Signals(13).YData = [-10 10 -10 10 -10 10 -10 10 -10 10 -10]
      | sbobj.Groups(3).Signals(14).Name = 'HwTqChB'
      | sbobj.Groups(3).Signals(14).XData = [0 1 1 2 2 3 3 4 4 5 5]
      | sbobj.Groups(3).Signals(14).YData = [-10 10 -10 10 -10 10 -10 10 -10 10 -10]
      | sbobj.Groups(3).TimeRange = [0 5]
      | sbobj.Groups(4).Name = 'HwTqA Qlfr Fault'
      | sbobj.Groups(4).Signals(1).Name = 'TqA'
      | sbobj.Groups(4).Signals(1).XData = [0 1 1 2 2 3 3 4 4 5]
      | sbobj.Groups(4).Signals(1).YData = [-10 10 -10 10 -10 10 -10 10 -10 10]
      | sbobj.Groups(4).Signals(2).Name = 'TqB'
      | sbobj.Groups(4).Signals(2).XData = [0 0.5 1 1 1.5 2 2 2.5 3 3.5 4 4 4.5 5]
      | sbobj.Groups(4).Signals(2).YData = [-10 10 9 -10 0 10 -10 0 0 0 10 -10 0 10]
      | sbobj.Groups(4).Signals(3).Name = 'TqC'
      | sbobj.Groups(4).Signals(3).XData = [0 1 1 2 2 3 3 4 4 5]
      | sbobj.Groups(4).Signals(3).YData = [-10 10 -10 10 -10 10 -10 10 -10 10]
      | sbobj.Groups(4).Signals(4).Name = 'TqD'
      | sbobj.Groups(4).Signals(4).XData = [0 1 1 2 2 3 3 4 4 5]
      | sbobj.Groups(4).Signals(4).YData = [-10 10 -10 10 -10 10 -10 10 -10 10]
      | sbobj.Groups(4).Signals(5).Name = 'TqARC'
      | sbobj.Groups(4).Signals(5).XData = [0 0.5 1 1 1.5 1.5 2 2 2.5 2.5 3 3.5 4 4 5]
      | sbobj.Groups(4).Signals(5).YData = [0 200 200 0 200 0 200 0 200 0 0 0 200 0 200]
      | sbobj.Groups(4).Signals(6).Name = 'TqAQlfr'
      | sbobj.Groups(4).Signals(6).XData = [0 0.5 0.5 1 1.5 1.5 2 2.5 2.75 2.75 3.5 3.5 4 4.5 5]
      | sbobj.Groups(4).Signals(6).YData = [1 1 2 2 2 1 1 1 1 2.05 2 1 1 1 1]
      | sbobj.Groups(4).Signals(7).Name = 'TqBRc'
      | sbobj.Groups(4).Signals(7).XData = [0 1 1 2 2 3 3 4 4 5]
      | sbobj.Groups(4).Signals(7).YData = [-1 255 -1 255 -1 255 -1 255 -1 255]
      | sbobj.Groups(4).Signals(8).Name = 'TqBQlfr'
      | sbobj.Groups(4).Signals(8).XData = [0 5]
      | sbobj.Groups(4).Signals(8).YData = [1 1]
      | sbobj.Groups(4).Signals(9).Name = 'TqCRC'
      | sbobj.Groups(4).Signals(9).XData = [0 1 1 2 2 3 3 4 4 5]
      | sbobj.Groups(4).Signals(9).YData = [-1 255 -1 255 -1 255 -1 255 -1 255]
      | sbobj.Groups(4).Signals(10).Name = 'TqCQlfr'
      | sbobj.Groups(4).Signals(10).XData = [0 5]
      | sbobj.Groups(4).Signals(10).YData = [1 1]
      | sbobj.Groups(4).Signals(11).Name = 'TqDRC'
      | sbobj.Groups(4).Signals(11).XData = [0 1 1 2 2 3 3 4 4 5]
      | sbobj.Groups(4).Signals(11).YData = [-1 255 -1 255 -1 255 -1 255 -1 255]
      | sbobj.Groups(4).Signals(12).Name = 'TqDQlfr'
      | sbobj.Groups(4).Signals(12).XData = [0 5]
      | sbobj.Groups(4).Signals(12).YData = [1 1]
      | sbobj.Groups(4).Signals(13).Name = 'HwTqChA'
      | sbobj.Groups(4).Signals(13).XData = [0 1 1 2 2 3 3 4 4 5 5]
      | sbobj.Groups(4).Signals(13).YData = [-10 10 -10 10 -10 10 -10 10 -10 10 -10]
      | sbobj.Groups(4).Signals(14).Name = 'HwTqChB'
      | sbobj.Groups(4).Signals(14).XData = [0 1 1 2 2 3 3 4 4 5 5]
      | sbobj.Groups(4).Signals(14).YData = [-10 10 -10 10 -10 10 -10 10 -10 10 -10]
      | sbobj.Groups(4).TimeRange = [0 5]
      | sbobj.Groups(5).Name = 'HwTqA Corrln and Avl Fault'
      | sbobj.Groups(5).Signals(1).Name = 'TqA'
      | sbobj.Groups(5).Signals(1).XData = [0 1 1 2 2 3 3 4 4 5]
      | sbobj.Groups(5).Signals(1).YData = [-10 10 -10 10 -10 10 -10 10 -10 10]
      | sbobj.Groups(5).Signals(2).Name = 'TqB'
      | sbobj.Groups(5).Signals(2).XData = [0 0.5 1 1 1.5 2 2 2.5 3 3.5 4 4 4.5 5]
      | sbobj.Groups(5).Signals(2).YData = [-10 -10 -9 -10 0 10 -10 0 0 0 10 -10 0 10]
      | sbobj.Groups(5).Signals(3).Name = 'TqC'
      | sbobj.Groups(5).Signals(3).XData = [0 1 1 2 2 3 3 4 4 5]
      | sbobj.Groups(5).Signals(3).YData = [-10 10 -10 10 -10 10 -10 10 -10 10]
      | sbobj.Groups(5).Signals(4).Name = 'TqD'
      | sbobj.Groups(5).Signals(4).XData = [0 1 1 2 2 3 3 4 4 5]
      | sbobj.Groups(5).Signals(4).YData = [-10 10 -10 10 -10 10 -10 10 -10 10]
      | sbobj.Groups(5).Signals(5).Name = 'TqARC'
      | sbobj.Groups(5).Signals(5).XData = [0 0.5 1 1 1.5 1.5 2 2 2.5 2.5 3 3.5 4 4 5]
      | sbobj.Groups(5).Signals(5).YData = [0 200 200 0 200 0 200 0 200 0 0 0 200 0 200]
      | sbobj.Groups(5).Signals(6).Name = 'TqAQlfr'
      | sbobj.Groups(5).Signals(6).XData = [0 5]
      | sbobj.Groups(5).Signals(6).YData = [1 1]
      | sbobj.Groups(5).Signals(7).Name = 'TqBRc'
      | sbobj.Groups(5).Signals(7).XData = [0 1 1 2 2 3 3 4 4 5]
      | sbobj.Groups(5).Signals(7).YData = [0 255 0 255 0 255 0 255 0 100]
      | sbobj.Groups(5).Signals(8).Name = 'TqBQlfr'
      | sbobj.Groups(5).Signals(8).XData = [0 5]
      | sbobj.Groups(5).Signals(8).YData = [1 1]
      | sbobj.Groups(5).Signals(9).Name = 'TqCRC'
      | sbobj.Groups(5).Signals(9).XData = [0 1 1 2 2 3 3 4 4 5]
      | sbobj.Groups(5).Signals(9).YData = [0 255 0 255 0 255 0 255 0 255]
      | sbobj.Groups(5).Signals(10).Name = 'TqCQlfr'
      | sbobj.Groups(5).Signals(10).XData = [0 5]
      | sbobj.Groups(5).Signals(10).YData = [1 1]
      | sbobj.Groups(5).Signals(11).Name = 'TqDRC'
      | sbobj.Groups(5).Signals(11).XData = [0 1 1 2 2 3 3 4 4 5]
      | sbobj.Groups(5).Signals(11).YData = [0 255 0 255 0 255 0 255 0 255]
      | sbobj.Groups(5).Signals(12).Name = 'TqDQlfr'
      | sbobj.Groups(5).Signals(12).XData = [0 5]
      | sbobj.Groups(5).Signals(12).YData = [1 1]
      | sbobj.Groups(5).Signals(13).Name = 'HwTqChA'
      | sbobj.Groups(5).Signals(13).XData = [0 1 1 2 2 3 3 4 4 5 5]
      | sbobj.Groups(5).Signals(13).YData = [-10 10 -10 10 -10 10 -10 10 -10 10 -10]
      | sbobj.Groups(5).Signals(14).Name = 'HwTqChB'
      | sbobj.Groups(5).Signals(14).XData = [0 1 1 2 2 3 3 4 4 5 5]
      | sbobj.Groups(5).Signals(14).YData = [-10 10 -10 10 -10 10 -10 10 -10 10 -10]
      | sbobj.Groups(5).TimeRange = [0 5]
  TqA : Outport  Tag=STV Outport
  TqB : Outport  Tag=STV Outport  Port=2
  TqC : Outport  Tag=STV Outport  Port=3
  TqD : Outport  Tag=STV Outport  Port=4
  TqARC : Outport  Tag=STV Outport  Port=5
  TqAQlfr : Outport  Tag=STV Outport  Port=6
  TqBRc : Outport  Tag=STV Outport  Port=7
  TqBQlfr : Outport  Tag=STV Outport  Port=8
  TqCRC : Outport  Tag=STV Outport  Port=9
  TqCQlfr : Outport  Tag=STV Outport  Port=10
  TqDRC : Outport  Tag=STV Outport  Port=11
  TqDQlfr : Outport  Tag=STV Outport  Port=12
  HwTqChA : Outport  Tag=STV Outport  Port=13
  HwTqChB : Outport  Tag=STV Outport  Port=14
  wires:
  FromWs/1 -> Demux/1
  Demux/1 -> TqA/1
  Demux/2 -> TqB/1
  Demux/3 -> TqC/1
  Demux/4 -> TqD/1
  Demux/5 -> TqARC/1
  Demux/6 -> TqAQlfr/1
  Demux/7 -> TqBRc/1
  Demux/8 -> TqBQlfr/1
  Demux/9 -> TqCRC/1
  Demux/10 -> TqCQlfr/1
  Demux/11 -> TqDRC/1
  Demux/12 -> TqDQlfr/1
  Demux/13 -> HwTqChA/1
  Demux/14 -> HwTqChB/1

== system ES229A_HwTqCorrln/HwTqCorrln/CopyRight2 ==

== system ES229A_HwTqCorrln/HwTqCorrln/HwTqCorrlnInit1 ==
  function : TriggerPort  TriggerType=function-call
  ChA Common Mode Compensation LPF Init : Subsystem  RequirementInfo="{'linktype_rmi_doors' '0000c477 (/ESG Group/FDD Module Requirements/EA4 Specific/ES229A_HwTqCorrln)' '#ES229A_127' 'true' 'REQ:  ES229A_127' '' } %GIDa_fa10f3eb_b802_42ab_867e_912847a702f5"
  ChA Steady State LPF Init : Fil/FilLpInit  RequirementInfo="{'linktype_rmi_doors' '0000c477 (/ESG Group/FDD Module Requirements/EA4 Specific/ES229A_HwTqCorrln)' '#ES229A_118' 'true' 'REQ:  ES229A_118' '' } %GIDa_846295c0_bf89_411d_975b_6a8975341813"  Ic=0  Ts=ARCHGLBPRM_100MILLISEC_SEC_F32  Freq=HwTqCorrlnChAStabStLpFilFrq  StVar=HwTqChAStabStLpFil
  ChA Transient Fault LPF Init : Subsystem  RequirementInfo={} %GIDa_9896831e_cdc4_4ce8_9cbe_99723e18516e
  ChB Common Mode Compensation LPF Init : Subsystem  RequirementInfo="{'linktype_rmi_doors' '0000c477 (/ESG Group/FDD Module Requirements/EA4 Specific/ES229A_HwTqCorrln)' '#ES229A_158' 'true' 'REQ:  ES229A_158' '' } %GIDa_d14b29dc_8e45_415f_ad1c_3d41ae1631eb"
  ChB Steady State LPF Init : Fil/FilLpInit  RequirementInfo="{'linktype_rmi_doors' '0000c477 (/ESG Group/FDD Module Requirements/EA4 Specific/ES229A_HwTqCorrln)' '#ES229A_132' 'true' 'REQ:  ES229A_132' '' } %GIDa_d0176d38_e187_447f_938f_447a9b0e6090"  Ic=0  Ts=ARCHGLBPRM_100MILLISEC_SEC_F32  Freq=HwTqCorrlnChBStabStLpFilFrq  StVar=HwTqChBStabStLpFil
  ChB Transient Fault LPF Init : Subsystem
  CopyRight2 : Subsystem  Description=|  mask(Copyright Information){none=on}
      | Copyright info block.                                               
      |                                                                     
      | Place copyright information at the top of every subsystem in design.
      mask prompts: none "No parameters"
      mask help: Place copyright information at the top of every subsystem in design.
      mask Display:
      | NxtrConf = 'Nexteer Confidential';
      | 
      | sys = bdroot; %handle for the current model ("system")
      | first = get_param(sys,'Created');
      | first = first(end-3:end);  %year is last four digits
      | 
      | last = get_param(sys,'LastModifiedDate');
      | if isempty(last)
      |     last = datestr(now,'yyyy');
      | else
      |     last = last(end-3:end);
      | end
      | 
      | if strcmp(first,last)
      |     fprintf('%s -- Copyright %s Nexteer',NxtrConf,first)
      | else
      |     fprintf('%s -- %s%s- %s Nexteer',NxtrConf,char(169),first,last)
      | end

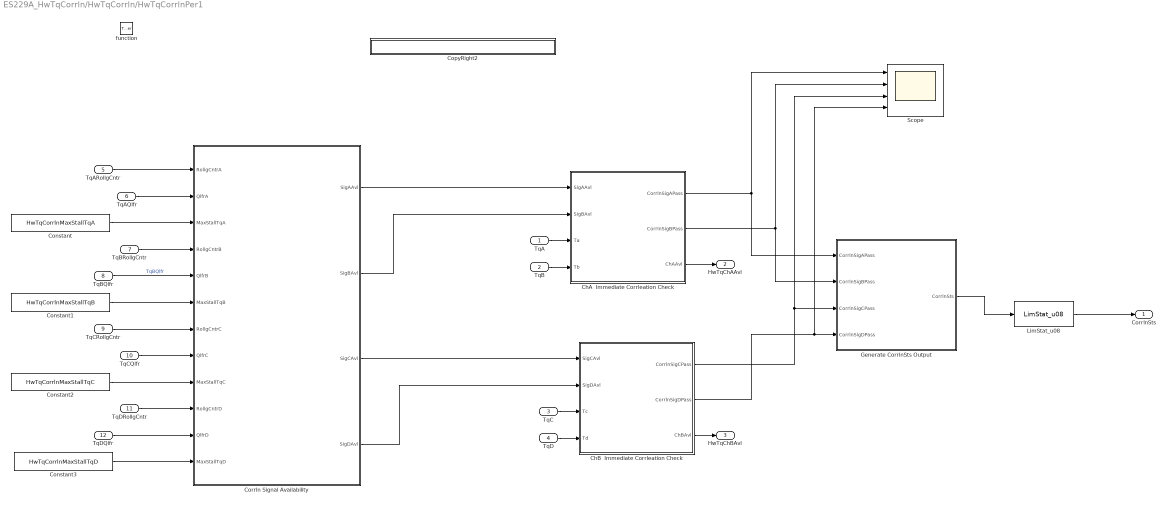
== system ES229A_HwTqCorrln/HwTqCorrln/HwTqCorrlnPer1 ==
  TqA : Inport
  TqB : Inport  Port=2
  TqC : Inport  Port=3
  TqD : Inport  Port=4
  TqARollgCntr : Inport  Port=5
  TqAQlfr : Inport  Port=6
  TqBRollgCntr : Inport  Port=7
  TqBQlfr : Inport  Port=8
  TqCRollgCntr : Inport  Port=9
  TqCQlfr : Inport  Port=10
  TqDRollgCntr : Inport  Port=11
  TqDQlfr : Inport  Port=12
  function : TriggerPort  TriggerType=function-call
  "ChA  Immediate Corrleation Check " : Subsystem  RequirementInfo="{'linktype_rmi_doors' '0000c477 (/ESG Group/FDD Module Requirements/EA4 Specific/ES229A_HwTqCorrln)' '#ES229A_105' 'true' 'REQ:  ES229A_105' '' ; 'linktype_rmi_doors' '0000c477 (/ESG Group/FDD Module Requirements/EA4 Specific/ES229A_HwTqCorrln)' '#ES229A_161' 'true' 'REQ:ES229A_161' '' } %GIDa_66f2ab77_874a_48f0_9064_4e411d222434"
  ChB  Immediate Corrleation Check : Subsystem  RequirementInfo="{'linktype_rmi_doors' '0000c477 (/ESG Group/FDD Module Requirements/EA4 Specific/ES229A_HwTqCorrln)' '#ES229A_114' 'true' 'REQ:  ES229A_114' '' ; 'linktype_rmi_doors' '0000c477 (/ESG Group/FDD Module Requirements/EA4 Specific/ES229A_HwTqCorrln)' '#ES229A_162' 'true' 'REQ:ES229A_162' '' } %GIDa_ea1f0d2b_0cb0_4dbc_8b11_9a4dafee9a0a"
  Constant : Constant  Value=HwTqCorrlnMaxStallTqA
  Constant1 : Constant  Value=HwTqCorrlnMaxStallTqB
  Constant2 : Constant  Value=HwTqCorrlnMaxStallTqC
  Constant3 : Constant  Value=HwTqCorrlnMaxStallTqD
  CopyRight2 : Subsystem  Description=|  mask(Copyright Information){none=on}
      | Copyright info block.                                               
      |                                                                     
      | Place copyright information at the top of every subsystem in design.
      mask prompts: none "No parameters"
      mask help: Place copyright information at the top of every subsystem in design.
      mask Display:
      | NxtrConf = 'Nexteer Confidential';
      | 
      | sys = bdroot; %handle for the current model ("system")
      | first = get_param(sys,'Created');
      | first = first(end-3:end);  %year is last four digits
      | 
      | last = get_param(sys,'LastModifiedDate');
      | if isempty(last)
      |     last = datestr(now,'yyyy');
      | else
      |     last = last(end-3:end);
      | end
      | 
      | if strcmp(first,last)
      |     fprintf('%s -- Copyright %s Nexteer',NxtrConf,first)
      | else
      |     fprintf('%s -- %s%s- %s Nexteer',NxtrConf,char(169),first,last)
      | end
  Corrln Signal Availability : Subsystem
  Generate CorrlnSts Output : Subsystem  RequirementInfo="{'linktype_rmi_doors' '0000c477 (/ESG Group/FDD Module Requirements/EA4 Specific/ES229A_HwTqCorrln)' '#ES229A_153' 'true' 'REQ:  ES229A_153' '' ; 'linktype_rmi_doors' '0000c477 (/ESG Group/FDD Module Requirements/EA4 Specific/ES229A_HwTqCorrln)' '#ES229A_154' 'true' 'REQ:  ES229A_154' '' } %GIDa_9802466a_586d_461c_9c14_ae6d761316a5"
  LimStat_u08 : NxtrLim/LimStat_u08  RequirementInfo="{'linktype_rmi_doors' '0000c477 (/ESG Group/FDD Module Requirements/EA4 Specific/ES229A_HwTqCorrln)' '#ES229A_160' 'true' 'REQ:  ES229A_160' '' } %GIDa_c10cda3e_44d1_4414_9c10_afc2301380c4"  LoLim=HWTQCORRLNSTSMINLMT_CNT_U08  HiLim=HWTQCORRLNSTSMAXLMT_CNT_U08
      settings: AttributesFormatString=|
      | Low Limit: %<LoLim>
      | High Limit:%<HiLim>
  Scope : Scope  NumInputPorts=4
      settings: TimeRange=auto  LimitDataPoints=on  MaxDataPoints=5000  SaveToWorkspace=off  YMin=-5~-5~-5~-5  YMax=5~5~5~5  SampleTime=-1
  CorrlnSts : Outport
  HwTqChAAvl : Outport  Port=2
  HwTqChBAvl : Outport  Port=3
  wires:
  TqA/1 -> "ChA  Immediate Corrleation Check "/3(Ta)
  TqD/1 -> ChB  Immediate Corrleation Check/4(Td)
  Corrln Signal Availability/1(SigAAvl) -> "ChA  Immediate Corrleation Check "/1(SigAAvl)
  TqAQlfr/1 -> Corrln Signal Availability/2(QlfrA)
  Constant/1 -> Corrln Signal Availability/3(MaxStallTqA)
  TqBRollgCntr/1 -> Corrln Signal Availability/4(RollgCntrB)
  TqBQlfr/1 -> Corrln Signal Availability/5(QlfrB)  "TqBQlfr"
  Constant1/1 -> Corrln Signal Availability/6(MaxStallTqB)
  TqCRollgCntr/1 -> Corrln Signal Availability/7(RollgCntrC)
  TqCQlfr/1 -> Corrln Signal Availability/8(QlfrC)
  Constant2/1 -> Corrln Signal Availability/9(MaxStallTqC)
  TqDRollgCntr/1 -> Corrln Signal Availability/10(RollgCntrD)
  TqDQlfr/1 -> Corrln Signal Availability/11(QlfrD)
  Constant3/1 -> Corrln Signal Availability/12(MaxStallTqD)
  TqARollgCntr/1 -> Corrln Signal Availability/1(RollgCntrA)
  TqC/1 -> ChB  Immediate Corrleation Check/3(Tc)
  Corrln Signal Availability/4(SigDAvl) -> ChB  Immediate Corrleation Check/2(SigDAvl)
  Corrln Signal Availability/3(SigCAvl) -> ChB  Immediate Corrleation Check/1(SigCAvl)
  TqB/1 -> "ChA  Immediate Corrleation Check "/4(Tb)
  "ChA  Immediate Corrleation Check "/1(CorrlnSigAPass) -> Scope/1, Generate CorrlnSts Output/1("CorrlnSigAPass ")
  "ChA  Immediate Corrleation Check "/2(CorrlnSigBPass) -> Scope/2, Generate CorrlnSts Output/2(CorrlnSigBPass)
  ChB  Immediate Corrleation Check/1(CorrlnSigCPass) -> Scope/3, Generate CorrlnSts Output/3(CorrlnSigCPass)
  ChB  Immediate Corrleation Check/2(CorrlnSigDPass) -> Scope/4, Generate CorrlnSts Output/4(CorrlnSigDPass)
  LimStat_u08/1 -> CorrlnSts/1
  Generate CorrlnSts Output/1(CorrlnSts) -> LimStat_u08/1
  Corrln Signal Availability/2(SigBAvl) -> "ChA  Immediate Corrleation Check "/2(SigBAvl)
  "ChA  Immediate Corrleation Check "/3(ChAAvl) -> HwTqChAAvl/1
  ChB  Immediate Corrleation Check/3(ChBAvl) -> HwTqChBAvl/1

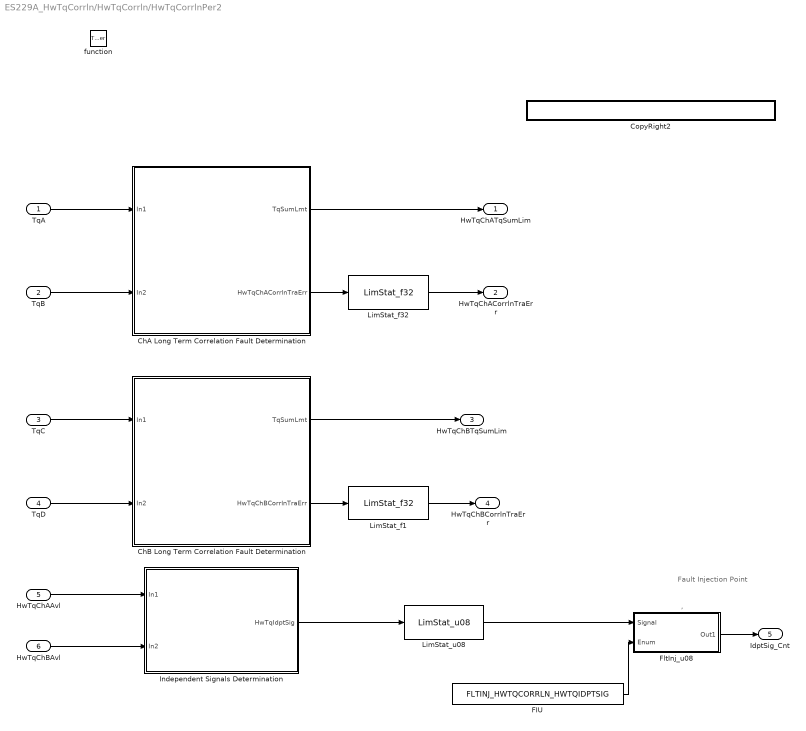
== system ES229A_HwTqCorrln/HwTqCorrln/HwTqCorrlnPer2 ==
  note: ,
  note: Fault
      | Injection
      | Point
  TqA : Inport
  TqB : Inport  Port=2
  TqC : Inport  Port=3
  TqD : Inport  Port=4
  HwTqChAAvl : Inport  Port=5
  HwTqChBAvl : Inport  Port=6
  function : TriggerPort  TriggerType=function-call
  ChA Long Term Correlation Fault Determination : Subsystem
  ChB Long Term Correlation Fault Determination : Subsystem
  CopyRight2 : Subsystem  Description=|  mask(Copyright Information){none=on}
      | Copyright info block.                                               
      |                                                                     
      | Place copyright information at the top of every subsystem in design.
      mask prompts: none "No parameters"
      mask help: Place copyright information at the top of every subsystem in design.
      mask Display:
      | NxtrConf = 'Nexteer Confidential';
      | 
      | sys = bdroot; %handle for the current model ("system")
      | first = get_param(sys,'Created');
      | first = first(end-3:end);  %year is last four digits
      | 
      | last = get_param(sys,'LastModifiedDate');
      | if isempty(last)
      |     last = datestr(now,'yyyy');
      | else
      |     last = last(end-3:end);
      | end
      | 
      | if strcmp(first,last)
      |     fprintf('%s -- Copyright %s Nexteer',NxtrConf,first)
      | else
      |     fprintf('%s -- %s%s- %s Nexteer',NxtrConf,char(169),first,last)
      | end
  FIU : Constant  RequirementInfo="{'linktype_rmi_doors' '0000c477 (/ESG Group/FDD Module Requirements/EA4 Specific/ES229A_HwTqCorrln)' '#ES229A_144' 'true' 'REQ:  ES229A_144' '' } %GIDa_e597b29f_e758_422e_89e1_29bd0aa49102"  Value=FLTINJ_HWTQCORRLN_HWTQIDPTSIG
  FltInj_u08 : Subsystem  RequirementInfo="{'linktype_rmi_doors' '0000c477 (/ESG Group/FDD Module Requirements/EA4 Specific/ES229A_HwTqCorrln)' '#ES229A_144' 'true' 'REQ:  ES229A_144' '' } %GIDa_dbaf9b57_221c_4539_ac07_ee929170e0c6"  TreatAsAtomicUnit=on  VariantControl=FltInj_sim  mask(Fault_Injection){}
      mask help: Fault Injection is a simulation only block for EA4 programs.
  Independent Signals Determination : Subsystem  RequirementInfo="{'linktype_rmi_doors' '0000c477 (/ESG Group/FDD Module Requirements/EA4 Specific/ES229A_HwTqCorrln)' '#ES229A_100' 'true' 'REQ:  ES229A_100' '' ; 'linktype_rmi_doors' '0000c477 (/ESG Group/FDD Module Requirements/EA4 Specific/ES229A_HwTqCorrln)' '#ES229A_101' 'true' 'REQ:  ES229A_101' '' ; 'linktype_rmi_doors' '0000c477 (/ESG Group/FDD Module Requirements/EA4 Specific/ES229A_HwTqCorrln)' '#ES229A_102' 'true' 'REQ:  ES229A_102' '' ; 'linktype_rmi_doors' '0000c477 (/ESG Group/FDD Module Requirements/EA4 Specific/ES229A_HwTqCorrln)' '#ES229A_77' 'true' 'REQ:  ES229A_77' '' } %GIDa_66a7ad0e_7467_4f6f_b9b9_69c5ff4bbc29"
  LimStat_f1 : NxtrLim/LimStat_f32  RequirementInfo={'linktype_rmi_doors' '0000c477 (/ESG Group/FDD Module Requirements/EA4 Specific/ES229A_HwTqCorrln)' '#ES229A_168' 'true' 'REQ: ES229A_168' '' } %GIDa_a3c93eb5_ef04_45cf_9007_842b96edfc27  LoLim=HwTqChBCorrlnTraErr.EngMin  HiLim=HwTqChBCorrlnTraErr.EngMax
      settings: AttributesFormatString=|
      | Low Limit: %<LoLim>
      | High Limit:%<HiLim>
  LimStat_f32 : NxtrLim/LimStat_f32  RequirementInfo={'linktype_rmi_doors' '0000c477 (/ESG Group/FDD Module Requirements/EA4 Specific/ES229A_HwTqCorrln)' '#ES229A_167' 'true' 'REQ: ES229A_167' '' } %GIDa_4f08ac36_53e5_4cf8_b115_169d7b64dba7  LoLim=HwTqChACorrlnTraErr.EngMin  HiLim=HwTqChACorrlnTraErr.EngMax
      settings: AttributesFormatString=|
      | Low Limit: %<LoLim>
      | High Limit:%<HiLim>
  LimStat_u08 : NxtrLim/LimStat_u08  RequirementInfo="{'linktype_rmi_doors' '0000c477 (/ESG Group/FDD Module Requirements/EA4 Specific/ES229A_HwTqCorrln)' '#ES229A_159' 'true' 'REQ:  ES229A_159' '' } %GIDa_3a38df1b_391b_4abd_b9b0_de9b11b58240"  LoLim=HWTQIDPDTSIGMINLMT_CNT_U08  HiLim=HWTQIDPDTSIGMAXLMT_CNT_U08
      settings: AttributesFormatString=|
      | Low Limit: %<LoLim>
      | High Limit:%<HiLim>
  HwTqChATqSumLim : Outport
  HwTqChACorrlnTraErr : Outport  Port=2
  HwTqChBTqSumLim : Outport  Port=3
  HwTqChBCorrlnTraErr : Outport  Port=4
  IdptSig_Cnt : Outport  Port=5
  wires:
  ChA Long Term Correlation Fault Determination/1(TqSumLmt) -> HwTqChATqSumLim/1
  TqA/1 -> ChA Long Term Correlation Fault Determination/1(In1)
  TqB/1 -> ChA Long Term Correlation Fault Determination/2(In2)
  TqC/1 -> ChB Long Term Correlation Fault Determination/1(In1)
  TqD/1 -> ChB Long Term Correlation Fault Determination/2(In2)
  ChB Long Term Correlation Fault Determination/1(TqSumLmt) -> HwTqChBTqSumLim/1
  Independent Signals Determination/1(HwTqIdptSig) -> LimStat_u08/1
  FIU/1 -> FltInj_u08/2(Enum)
  FltInj_u08/1(Out1) -> IdptSig_Cnt/1
  LimStat_u08/1 -> FltInj_u08/1(Signal)
  HwTqChBAvl/1 -> Independent Signals Determination/2(In2)
  HwTqChAAvl/1 -> Independent Signals Determination/1(In1)
  ChA Long Term Correlation Fault Determination/2(HwTqChACorrlnTraErr) -> LimStat_f32/1
  ChB Long Term Correlation Fault Determination/2(HwTqChBCorrlnTraErr) -> LimStat_f1/1
  LimStat_f32/1 -> HwTqChACorrlnTraErr/1
  LimStat_f1/1 -> HwTqChBCorrlnTraErr/1

== system ES229A_HwTqCorrln/HwTqCorrln/HwTqCorrlnPer3 ==
  HwTqChA : Inport
  HwTqChATqSumLmt : Inport  Port=2
  HwTqChB : Inport  Port=3
  HwTqChBTqSumLmt : Inport  Port=4
  function : TriggerPort  TriggerType=function-call
  ChA Long Term Offset Compensation : Subsystem  RequirementInfo={'linktype_rmi_doors' '0000c477 (/ESG Group/FDD Module Requirements/EA4 Specific/ES229A_HwTqCorrln)' '#ES229A_118' 'true' 'REQ:ES229A_118' '' ; 'linktype_rmi_doors' '0000c477 (/ESG Group/FDD Module Requirements/EA4 Specific/ES229A_HwTqCorrln)' '#ES229A_163' 'true' 'REQ:ES229A_163' '' } %GIDa_99ed9894_8645_4b4b_b80c_34beb74593d1
  ChB Long Term Offset Compensation : Subsystem  RequirementInfo={'linktype_rmi_doors' '0000c477 (/ESG Group/FDD Module Requirements/EA4 Specific/ES229A_HwTqCorrln)' '#ES229A_132' 'true' 'REQ:ES229A_132' '' ; 'linktype_rmi_doors' '0000c477 (/ESG Group/FDD Module Requirements/EA4 Specific/ES229A_HwTqCorrln)' '#ES229A_164' 'true' 'REQ:ES229A_164' '' } %GIDa_64731a86_1980_4f3b_b7a4_5dc50a4d55b5
  CopyRight2 : Subsystem  Description=|  mask(Copyright Information){none=on}
      | Copyright info block.                                               
      |                                                                     
      | Place copyright information at the top of every subsystem in design.
      mask prompts: none "No parameters"
      mask help: Place copyright information at the top of every subsystem in design.
      mask Display:
      | NxtrConf = 'Nexteer Confidential';
      | 
      | sys = bdroot; %handle for the current model ("system")
      | first = get_param(sys,'Created');
      | first = first(end-3:end);  %year is last four digits
      | 
      | last = get_param(sys,'LastModifiedDate');
      | if isempty(last)
      |     last = datestr(now,'yyyy');
      | else
      |     last = last(end-3:end);
      | end
      | 
      | if strcmp(first,last)
      |     fprintf('%s -- Copyright %s Nexteer',NxtrConf,first)
      | else
      |     fprintf('%s -- %s%s- %s Nexteer',NxtrConf,char(169),first,last)
      | end
  wires:
  HwTqChATqSumLmt/1 -> ChA Long Term Offset Compensation/2(TqSumLmt)
  HwTqChA/1 -> ChA Long Term Offset Compensation/1(Hw Tq)
  HwTqChBTqSumLmt/1 -> ChB Long Term Offset Compensation/2(TqSumLmt)
  HwTqChB/1 -> ChB Long Term Offset Compensation/1(Hw Tq)

== system ES229A_HwTqCorrln/HwTqCorrln/HwTqCorrlnInit1/ChA Common Mode Compensation LPF Init ==
  "ChA CMC LPF Init - Fc " : Fil/FilLpInit  Priority=1  Ic=0  Ts=ARCHGLBPRM_100MILLISEC_SEC_F32  Freq=HwTqCorrlnChACmnModCmpLpFilFrq  StVar=HwTqChACmnModCmpLpFil
      settings: AttributesFormatString=Priority: %<Priority>
  CopyRight2 : Subsystem  Description=|  mask(Copyright Information){none=on}
      | Copyright info block.                                               
      |                                                                     
      | Place copyright information at the top of every subsystem in design.
      mask prompts: none "No parameters"
      mask help: Place copyright information at the top of every subsystem in design.
      mask Display:
      | NxtrConf = 'Nexteer Confidential';
      | 
      | sys = bdroot; %handle for the current model ("system")
      | first = get_param(sys,'Created');
      | first = first(end-3:end);  %year is last four digits
      | 
      | last = get_param(sys,'LastModifiedDate');
      | if isempty(last)
      |     last = datestr(now,'yyyy');
      | else
      |     last = last(end-3:end);
      | end
      | 
      | if strcmp(first,last)
      |     fprintf('%s -- Copyright %s Nexteer',NxtrConf,first)
      | else
      |     fprintf('%s -- %s%s- %s Nexteer',NxtrConf,char(169),first,last)
      | end
  Data Store Read Sv NVM Shadowed RAM : DataStoreRead  DataStoreName=HwTqChACmnModCmpLpFilSt
  Data Store Write1 : DataStoreWrite  Priority=2  DataStoreName=HwTqChACmnModCmpLpFil  DataStoreElements=HwTqChACmnModCmpLpFil.FilSt
      settings: AttributesFormatString=Priority: %<Priority>
  wires:
  Data Store Read Sv NVM Shadowed RAM/1 -> Data Store Write1/1

== system ES229A_HwTqCorrln/HwTqCorrln/HwTqCorrlnInit1/ChA Transient Fault LPF Init ==
  Constant : Constant  Value=0  OutDataTypeStr=single
  CopyRight2 : Subsystem  Description=|  mask(Copyright Information){none=on}
      | Copyright info block.                                               
      |                                                                     
      | Place copyright information at the top of every subsystem in design.
      mask prompts: none "No parameters"
      mask help: Place copyright information at the top of every subsystem in design.
      mask Display:
      | NxtrConf = 'Nexteer Confidential';
      | 
      | sys = bdroot; %handle for the current model ("system")
      | first = get_param(sys,'Created');
      | first = first(end-3:end);  %year is last four digits
      | 
      | last = get_param(sys,'LastModifiedDate');
      | if isempty(last)
      |     last = datestr(now,'yyyy');
      | else
      |     last = last(end-3:end);
      | end
      | 
      | if strcmp(first,last)
      |     fprintf('%s -- Copyright %s Nexteer',NxtrConf,first)
      | else
      |     fprintf('%s -- %s%s- %s Nexteer',NxtrConf,char(169),first,last)
      | end
  Data Store Write1 : DataStoreWrite  DataStoreName=HwTqChATraLpFil  DataStoreElements=HwTqChATraLpFil.FilSt
  wires:
  Constant/1 -> Data Store Write1/1

== system ES229A_HwTqCorrln/HwTqCorrln/HwTqCorrlnInit1/ChB Common Mode Compensation LPF Init ==
  ChB CMC LPF Init - Fc : Fil/FilLpInit  Priority=1  Ic=0  Ts=ARCHGLBPRM_100MILLISEC_SEC_F32  Freq=HwTqCorrlnChBCmnModCmpLpFilFrq  StVar=HwTqChBCmnModCmpLpFil
      settings: AttributesFormatString=Priority: %<Priority>
  CopyRight2 : Subsystem  Description=|  mask(Copyright Information){none=on}
      | Copyright info block.                                               
      |                                                                     
      | Place copyright information at the top of every subsystem in design.
      mask prompts: none "No parameters"
      mask help: Place copyright information at the top of every subsystem in design.
      mask Display:
      | NxtrConf = 'Nexteer Confidential';
      | 
      | sys = bdroot; %handle for the current model ("system")
      | first = get_param(sys,'Created');
      | first = first(end-3:end);  %year is last four digits
      | 
      | last = get_param(sys,'LastModifiedDate');
      | if isempty(last)
      |     last = datestr(now,'yyyy');
      | else
      |     last = last(end-3:end);
      | end
      | 
      | if strcmp(first,last)
      |     fprintf('%s -- Copyright %s Nexteer',NxtrConf,first)
      | else
      |     fprintf('%s -- %s%s- %s Nexteer',NxtrConf,char(169),first,last)
      | end
  Data Store Read Sv NVM Shadowed RAM : DataStoreRead  DataStoreName=HwTqChBCmnModCmpLpFilSt
  Data Store Write1 : DataStoreWrite  Priority=2  DataStoreName=HwTqChBCmnModCmpLpFil  DataStoreElements=HwTqChBCmnModCmpLpFil.FilSt
      settings: AttributesFormatString=Priority: %<Priority>
  wires:
  Data Store Read Sv NVM Shadowed RAM/1 -> Data Store Write1/1

== system ES229A_HwTqCorrln/HwTqCorrln/HwTqCorrlnInit1/ChB Transient Fault LPF Init ==
  Constant1 : Constant  Value=0  OutDataTypeStr=single
  CopyRight2 : Subsystem  Description=|  mask(Copyright Information){none=on}
      | Copyright info block.                                               
      |                                                                     
      | Place copyright information at the top of every subsystem in design.
      mask prompts: none "No parameters"
      mask help: Place copyright information at the top of every subsystem in design.
      mask Display:
      | NxtrConf = 'Nexteer Confidential';
      | 
      | sys = bdroot; %handle for the current model ("system")
      | first = get_param(sys,'Created');
      | first = first(end-3:end);  %year is last four digits
      | 
      | last = get_param(sys,'LastModifiedDate');
      | if isempty(last)
      |     last = datestr(now,'yyyy');
      | else
      |     last = last(end-3:end);
      | end
      | 
      | if strcmp(first,last)
      |     fprintf('%s -- Copyright %s Nexteer',NxtrConf,first)
      | else
      |     fprintf('%s -- %s%s- %s Nexteer',NxtrConf,char(169),first,last)
      | end
  Data Store Write : DataStoreWrite  DataStoreName=HwTqChBTraLpFil  DataStoreElements=HwTqChBTraLpFil.FilSt
  wires:
  Constant1/1 -> Data Store Write/1

== system ES229A_HwTqCorrln/HwTqCorrln/HwTqCorrlnInit1/CopyRight2 ==

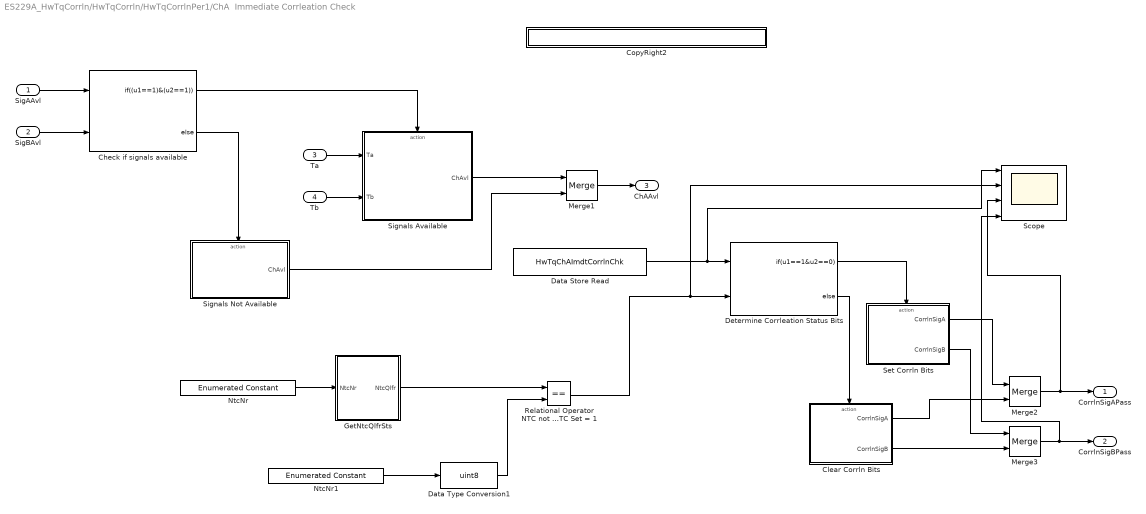
== system ES229A_HwTqCorrln/HwTqCorrln/HwTqCorrlnPer1/ChA  Immediate Corrleation Check  ==
  SigAAvl : Inport
  SigBAvl : Inport  Port=2
  Ta : Inport  Port=3
  Tb : Inport  Port=4
  Check if signals available : If  NumInputs=2  IfExpression=(u1==1)&(u2==1)
  Clear Corrln Bits : Subsystem  TreatAsAtomicUnit=on
  CopyRight2 : Subsystem  Description=|  mask(Copyright Information){none=on}
      | Copyright info block.                                               
      |                                                                     
      | Place copyright information at the top of every subsystem in design.
      mask prompts: none "No parameters"
      mask help: Place copyright information at the top of every subsystem in design.
      mask Display:
      | NxtrConf = 'Nexteer Confidential';
      | 
      | sys = bdroot; %handle for the current model ("system")
      | first = get_param(sys,'Created');
      | first = first(end-3:end);  %year is last four digits
      | 
      | last = get_param(sys,'LastModifiedDate');
      | if isempty(last)
      |     last = datestr(now,'yyyy');
      | else
      |     last = last(end-3:end);
      | end
      | 
      | if strcmp(first,last)
      |     fprintf('%s -- Copyright %s Nexteer',NxtrConf,first)
      | else
      |     fprintf('%s -- %s%s- %s Nexteer',NxtrConf,char(169),first,last)
      | end
  Data Store Read : DataStoreRead  DataStoreName=HwTqChAImdtCorrlnChk
  Data Type Conversion1 : DataTypeConversion  OutDataTypeStr=uint8
  Determine Corrleation Status Bits : If  NumInputs=2  IfExpression=u1==1&u2==0
  GetNtcQlfrSts : Subsystem  RequirementInfo={} %GIDa_3bd1d81f_a3f8_4a77_b2dd_26dc6ac4a557  TreatAsAtomicUnit=on  mask(GetNTC){}
      mask help: GetNTC library block
      settings: RTWSystemCode=Inline
  Merge1 : Merge
  Merge2 : Merge
  Merge3 : Merge
  NtcNr : simulink/Sources/Enumerated Constant  OutDataTypeStr=Enum: NtcNr1  Value=NtcNr1.NTCNR_0X070  SampleTime=inf
  NtcNr1 : simulink/Sources/Enumerated Constant  OutDataTypeStr=Enum: SigQlfr1  Value=SigQlfr1.SIGQLFR_FAILD  SampleTime=inf
  "Relational Operator NTC not Set = 0, NTC Set = 1" : RelationalOperator  Operator===  OutDataTypeStr=boolean
  Scope : Scope  NumInputPorts=4
      settings: TimeRange=auto  MaxDataPoints=5000  SaveToWorkspace=off  SaveName=ScopeData2  YMin=-5~-5~-5~-5  YMax=5~5~5~5  SampleTime=-1
  Set Corrln Bits : Subsystem  TreatAsAtomicUnit=on
  Signals Available : Subsystem  RequirementInfo={'linktype_rmi_doors' '0000c477 (/ESG Group/FDD Module Requirements/EA4 Specific/ES229A_HwTqCorrln)' '#ES229A_105' 'true' 'REQ:ES229A_105' '' } %GIDa_62ee8cc3_6675_413c_96ca_1fba29cca284  TreatAsAtomicUnit=on
  Signals Not Available : Subsystem  RequirementInfo={'linktype_rmi_doors' '0000c477 (/ESG Group/FDD Module Requirements/EA4 Specific/ES229A_HwTqCorrln)' '#ES229A_161' 'true' 'REQ:ES229A_161' '' } %GIDa_5b6bbcaa_26b5_4380_8331_3933f278185f  TreatAsAtomicUnit=on
  CorrlnSigAPass : Outport
  CorrlnSigBPass : Outport  Port=2
  ChAAvl : Outport  Port=3
  wires:
  Ta/1 -> Signals Available/1(Ta)
  Tb/1 -> Signals Available/2(Tb)
  Merge3/1 -> Scope/4, CorrlnSigBPass/1
  Determine Corrleation Status Bits/2 -> Clear Corrln Bits/Action
  Determine Corrleation Status Bits/1 -> Set Corrln Bits/Action
  Set Corrln Bits/1(CorrlnSigA) -> Merge2/1
  Clear Corrln Bits/1(CorrlnSigA) -> Merge2/2
  Clear Corrln Bits/2(CorrlnSigB) -> Merge3/2
  NtcNr/1 -> GetNtcQlfrSts/1(NtcNr)
  GetNtcQlfrSts/1(NtcQlfr) -> "Relational Operator NTC not Set = 0, NTC Set = 1"/1
  Check if signals available/1 -> Signals Available/Action
  Check if signals available/2 -> Signals Not Available/Action
  Data Store Read/1 -> Scope/1, Determine Corrleation Status Bits/1
  SigAAvl/1 -> Check if signals available/1
  SigBAvl/1 -> Check if signals available/2
  Merge2/1 -> Scope/3, CorrlnSigAPass/1
  Set Corrln Bits/2(CorrlnSigB) -> Merge3/1
  Data Type Conversion1/1 -> "Relational Operator NTC not Set = 0, NTC Set = 1"/2
  NtcNr1/1 -> Data Type Conversion1/1
  "Relational Operator NTC not Set = 0, NTC Set = 1"/1 -> Scope/2, Determine Corrleation Status Bits/2
  Signals Available/1(ChAvl) -> Merge1/1
  Signals Not Available/1(ChAvl) -> Merge1/2
  Merge1/1 -> ChAAvl/1
